simulink model "Quadcopter"  (R2018a)
settings: Solver=VariableStepAuto  StartTime=0.0  StopTime=30  RelTol=1e-3
undefined symbols (not defined in the file): sigbuilder_block
libraries: simulink x5
settings Model: Creator=Admin  LastModifiedBy=Admin

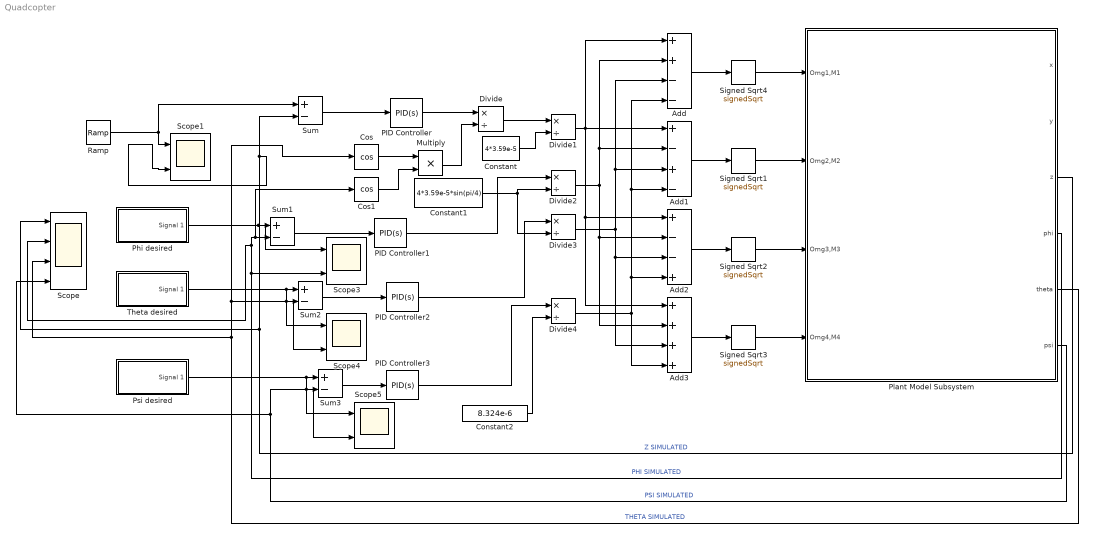
== system Quadcopter ==
  Add : Sum  Inputs=++--
  Add1 : Sum  Inputs=+-+-
  Add2 : Sum  Inputs=+--+
  Add3 : Sum  Inputs=++++
  Constant : Constant  Value=4*3.59e-5
  Constant1 : Constant  Value=4*3.59e-5*sin(pi/4)
  Constant2 : Constant  Value=8.324e-6
  Cos : Trigonometry  Operator=cos
  Cos1 : Trigonometry  Operator=cos
  Divide{,1..4} (5 alike) : Product  Inputs=*/
  Multiply : Product
  PID Controller : simulink/Continuous/PID Controller  Controller=PID  TimeDomain=Continuous-time  SampleTime=-1  IntegratorMethod=Forward Euler  FilterMethod=Forward Euler  Form=Parallel  UseFilter=on  ControllerParametersSource=internal  P=5.605  I=1.3  D=1.3  N=100  InitialConditionSource=internal  InitialConditionForIntegrator=0  InitialConditionForFilter=0  ExternalReset=none  LimitOutput=off  UpperSaturationLimit=inf  LowerSaturationLimit=-inf  LinearizeAsGain=on  AntiWindupMode=none  Kb=1  TrackingMode=off  Kt=1  PParamMin=[]  PParamMax=[]  IParamMin=[]  IParamMax=[]  DParamMin=[]  DParamMax=[]  NParamMin=[]  NParamMax=[]  KbParamMin=[]  KbParamMax=[]  KtParamMin=[]  KtParamMax=[]  POutMin=[]  POutMax=[]  IOutMin=[]  IOutMax=[]  DOutMin=[]  DOutMax=[]  NOutMin=[]  NOutMax=[]  KbOutMin=[]  KbOutMax=[]  KtOutMin=[]  KtOutMax=[]  IntegratorOutMin=[]  IntegratorOutMax=[]  FilterOutMin=[]  FilterOutMax=[]  SumOutMin=[]  SumOutMax=[]  SumI1OutMin=[]  SumI1OutMax=[]  SumI2OutMin=[]  SumI2OutMax=[]  SumI3OutMin=[]  SumI3OutMax=[]  SumDOutMin=[]  SumDOutMax=[]  SaturationOutMin=[]  SaturationOutMax=[]  IntegratorContinuousStateAttributes=''  IntegratorStateMustResolveToSignalObject=off  IntegratorRTWStateStorageClass=Auto  FilterContinuousStateAttributes=''  FilterStateMustResolveToSignalObject=off  FilterRTWStateStorageClass=Auto  DifferentiatorICPrevScaledInput=0  DifferentiatorOutMin=[]  DifferentiatorOutMax=[]  FilterDiffOutCoefMin=[]  FilterDiffOutCoefMax=[]  SumDenOutMin=[]  SumDenOutMax=[]  SumNumOutMin=[]  SumNumOutMax=[]  ReciprocalOutMin=[]  ReciprocalOutMax=[]  DivideOutMin=[]  DivideOutMax=[]  TunerSelectOption=Transfer Function Based (PID Tuner App)
  PID Controller1 : simulink/Continuous/PID Controller  Controller=PID  TimeDomain=Continuous-time  SampleTime=-1  IntegratorMethod=Forward Euler  FilterMethod=Forward Euler  Form=Parallel  UseFilter=on  ControllerParametersSource=internal  P=0.006  I=0.0001  D=0.2  N=100  InitialConditionSource=internal  InitialConditionForIntegrator=0  InitialConditionForFilter=0  ExternalReset=none  LimitOutput=off  UpperSaturationLimit=inf  LowerSaturationLimit=-inf  LinearizeAsGain=on  AntiWindupMode=none  Kb=1  TrackingMode=off  Kt=1  PParamMin=[]  PParamMax=[]  IParamMin=[]  IParamMax=[]  DParamMin=[]  DParamMax=[]  NParamMin=[]  NParamMax=[]  KbParamMin=[]  KbParamMax=[]  KtParamMin=[]  KtParamMax=[]  POutMin=[]  POutMax=[]  IOutMin=[]  IOutMax=[]  DOutMin=[]  DOutMax=[]  NOutMin=[]  NOutMax=[]  KbOutMin=[]  KbOutMax=[]  KtOutMin=[]  KtOutMax=[]  IntegratorOutMin=[]  IntegratorOutMax=[]  FilterOutMin=[]  FilterOutMax=[]  SumOutMin=[]  SumOutMax=[]  SumI1OutMin=[]  SumI1OutMax=[]  SumI2OutMin=[]  SumI2OutMax=[]  SumI3OutMin=[]  SumI3OutMax=[]  SumDOutMin=[]  SumDOutMax=[]  SaturationOutMin=[]  SaturationOutMax=[]  IntegratorContinuousStateAttributes=''  IntegratorStateMustResolveToSignalObject=off  IntegratorRTWStateStorageClass=Auto  FilterContinuousStateAttributes=''  FilterStateMustResolveToSignalObject=off  FilterRTWStateStorageClass=Auto  DifferentiatorICPrevScaledInput=0  DifferentiatorOutMin=[]  DifferentiatorOutMax=[]  FilterDiffOutCoefMin=[]  FilterDiffOutCoefMax=[]  SumDenOutMin=[]  SumDenOutMax=[]  SumNumOutMin=[]  SumNumOutMax=[]  ReciprocalOutMin=[]  ReciprocalOutMax=[]  DivideOutMin=[]  DivideOutMax=[]  TunerSelectOption=Transfer Function Based (PID Tuner App)
  PID Controller2 : simulink/Continuous/PID Controller  Controller=PID  TimeDomain=Continuous-time  SampleTime=-1  IntegratorMethod=Forward Euler  FilterMethod=Forward Euler  Form=Parallel  UseFilter=on  ControllerParametersSource=internal  P=0.006  I=0.0001  D=0.2  N=100  InitialConditionSource=internal  InitialConditionForIntegrator=0  InitialConditionForFilter=0  ExternalReset=none  LimitOutput=off  UpperSaturationLimit=inf  LowerSaturationLimit=-inf  LinearizeAsGain=on  AntiWindupMode=none  Kb=1  TrackingMode=off  Kt=1  PParamMin=[]  PParamMax=[]  IParamMin=[]  IParamMax=[]  DParamMin=[]  DParamMax=[]  NParamMin=[]  NParamMax=[]  KbParamMin=[]  KbParamMax=[]  KtParamMin=[]  KtParamMax=[]  POutMin=[]  POutMax=[]  IOutMin=[]  IOutMax=[]  DOutMin=[]  DOutMax=[]  NOutMin=[]  NOutMax=[]  KbOutMin=[]  KbOutMax=[]  KtOutMin=[]  KtOutMax=[]  IntegratorOutMin=[]  IntegratorOutMax=[]  FilterOutMin=[]  FilterOutMax=[]  SumOutMin=[]  SumOutMax=[]  SumI1OutMin=[]  SumI1OutMax=[]  SumI2OutMin=[]  SumI2OutMax=[]  SumI3OutMin=[]  SumI3OutMax=[]  SumDOutMin=[]  SumDOutMax=[]  SaturationOutMin=[]  SaturationOutMax=[]  IntegratorContinuousStateAttributes=''  IntegratorStateMustResolveToSignalObject=off  IntegratorRTWStateStorageClass=Auto  FilterContinuousStateAttributes=''  FilterStateMustResolveToSignalObject=off  FilterRTWStateStorageClass=Auto  DifferentiatorICPrevScaledInput=0  DifferentiatorOutMin=[]  DifferentiatorOutMax=[]  FilterDiffOutCoefMin=[]  FilterDiffOutCoefMax=[]  SumDenOutMin=[]  SumDenOutMax=[]  SumNumOutMin=[]  SumNumOutMax=[]  ReciprocalOutMin=[]  ReciprocalOutMax=[]  DivideOutMin=[]  DivideOutMax=[]  TunerSelectOption=Transfer Function Based (PID Tuner App)
  PID Controller3 : simulink/Continuous/PID Controller  Controller=PID  TimeDomain=Continuous-time  SampleTime=-1  IntegratorMethod=Forward Euler  FilterMethod=Forward Euler  Form=Parallel  UseFilter=on  ControllerParametersSource=internal  P=0.09  I=0.005  D=0.07  N=100  InitialConditionSource=internal  InitialConditionForIntegrator=0  InitialConditionForFilter=0  ExternalReset=none  LimitOutput=off  UpperSaturationLimit=inf  LowerSaturationLimit=-inf  LinearizeAsGain=on  AntiWindupMode=none  Kb=1  TrackingMode=off  Kt=1  PParamMin=[]  PParamMax=[]  IParamMin=[]  IParamMax=[]  DParamMin=[]  DParamMax=[]  NParamMin=[]  NParamMax=[]  KbParamMin=[]  KbParamMax=[]  KtParamMin=[]  KtParamMax=[]  POutMin=[]  POutMax=[]  IOutMin=[]  IOutMax=[]  DOutMin=[]  DOutMax=[]  NOutMin=[]  NOutMax=[]  KbOutMin=[]  KbOutMax=[]  KtOutMin=[]  KtOutMax=[]  IntegratorOutMin=[]  IntegratorOutMax=[]  FilterOutMin=[]  FilterOutMax=[]  SumOutMin=[]  SumOutMax=[]  SumI1OutMin=[]  SumI1OutMax=[]  SumI2OutMin=[]  SumI2OutMax=[]  SumI3OutMin=[]  SumI3OutMax=[]  SumDOutMin=[]  SumDOutMax=[]  SaturationOutMin=[]  SaturationOutMax=[]  IntegratorContinuousStateAttributes=''  IntegratorStateMustResolveToSignalObject=off  IntegratorRTWStateStorageClass=Auto  FilterContinuousStateAttributes=''  FilterStateMustResolveToSignalObject=off  FilterRTWStateStorageClass=Auto  DifferentiatorICPrevScaledInput=0  DifferentiatorOutMin=[]  DifferentiatorOutMax=[]  FilterDiffOutCoefMin=[]  FilterDiffOutCoefMax=[]  SumDenOutMin=[]  SumDenOutMax=[]  SumNumOutMin=[]  SumNumOutMax=[]  ReciprocalOutMin=[]  ReciprocalOutMax=[]  DivideOutMin=[]  DivideOutMax=[]  TunerSelectOption=Transfer Function Based (PID Tuner App)
  Phi desired : Subsystem  Tag=STV Subsys  LoadFcn=sigbuilder_block('load');  StartFcn=sigbuilder_block('start');  StopFcn=sigbuilder_block('stop');  ClipboardFcn=sigbuilder_block('clipboard');  mask(Sigbuilder block){tuvar=[0:10]}
      mask help: Simulink:masks:SigbuilderBlock_MD
      mask init:
      | if ~strcmp(get_param(bdroot(gcbh),'SimulationStatus'),'stopped') tuvar = sigbuilder_block('maskInit'); end
      settings: CopyFcn=sigbuilder_block('copy');  DeleteFcn=sigbuilder_block('delete');  ModelCloseFcn=sigbuilder_block('modelClose');  PreSaveFcn=sigbuilder_block('preSave');  PauseFcn=sigbuilder_block('pause');  ContinueFcn=sigbuilder_block('continue');  NameChangeFcn=sigbuilder_block('namechange');  OpenFcn=sigbuilder_block('open',[426.6 123.6 550.8 400.2 ]);  CloseFcn=sigbuilder_block('close');
      mask Display: plot(0, 0, 100, 100,[2, 2, 32, 32, 2], [68, 8, 8, 68, 68],[32, 2], [38, 38], [32, 19, 2],[53, 60, 44], [32, 17, 17, 2],[16, 16, 31, 31]);txt = getActiveGroup(gcbh);text(2, 100, txt,'verticalAlignment', 'top');
  Plant Model Subsystem : Subsystem
  Psi desired : Subsystem  Tag=STV Subsys  LoadFcn=sigbuilder_block('load');  StartFcn=sigbuilder_block('start');  StopFcn=sigbuilder_block('stop');  ClipboardFcn=sigbuilder_block('clipboard');  mask(Sigbuilder block){tuvar=[0:10]}
      mask help: Simulink:masks:SigbuilderBlock_MD
      mask init:
      | if ~strcmp(get_param(bdroot(gcbh),'SimulationStatus'),'stopped') tuvar = sigbuilder_block('maskInit'); end
      settings: CopyFcn=sigbuilder_block('copy');  DeleteFcn=sigbuilder_block('delete');  ModelCloseFcn=sigbuilder_block('modelClose');  PreSaveFcn=sigbuilder_block('preSave');  PauseFcn=sigbuilder_block('pause');  ContinueFcn=sigbuilder_block('continue');  NameChangeFcn=sigbuilder_block('namechange');  OpenFcn=sigbuilder_block('open',[426.6 123.6 550.8 400.2 ]);  CloseFcn=sigbuilder_block('close');
      mask Display: plot(0, 0, 100, 100,[2, 2, 32, 32, 2], [68, 8, 8, 68, 68],[32, 2], [38, 38], [32, 19, 2],[53, 60, 44], [32, 17, 17, 2],[16, 16, 31, 31]);txt = getActiveGroup(gcbh);text(2, 100, txt,'verticalAlignment', 'top');
  Ramp : simulink/Sources/Ramp  slope=1.5  start=0  InitialOutput=0
  Scope : Scope  NumInputPorts=4
  Scope{1,3..5} (4 alike) : Scope  NumInputPorts=2
  Signed Sqrt{1..4} (4 alike) : Sqrt  Operator=signedSqrt  SaturateOnIntegerOverflow=on
  Sum{,1..3} (4 alike) : Sum  Inputs=+-
  Theta desired : Subsystem  Tag=STV Subsys  LoadFcn=sigbuilder_block('load');  StartFcn=sigbuilder_block('start');  StopFcn=sigbuilder_block('stop');  ClipboardFcn=sigbuilder_block('clipboard');  mask(Sigbuilder block){tuvar=[0:10]}
      mask help: Simulink:masks:SigbuilderBlock_MD
      mask init:
      | if ~strcmp(get_param(bdroot(gcbh),'SimulationStatus'),'stopped') tuvar = sigbuilder_block('maskInit'); end
      settings: CopyFcn=sigbuilder_block('copy');  DeleteFcn=sigbuilder_block('delete');  ModelCloseFcn=sigbuilder_block('modelClose');  PreSaveFcn=sigbuilder_block('preSave');  PauseFcn=sigbuilder_block('pause');  ContinueFcn=sigbuilder_block('continue');  NameChangeFcn=sigbuilder_block('namechange');  OpenFcn=sigbuilder_block('open',[426.6 123.6 550.8 400.2 ]);  CloseFcn=sigbuilder_block('close');
      mask Display: plot(0, 0, 100, 100,[2, 2, 32, 32, 2], [68, 8, 8, 68, 68],[32, 2], [38, 38], [32, 19, 2],[53, 60, 44], [32, 17, 17, 2],[16, 16, 31, 31]);txt = getActiveGroup(gcbh);text(2, 100, txt,'verticalAlignment', 'top');
  wires:
  Sum/1 -> PID Controller/1
  PID Controller/1 -> Divide/1
  Multiply/1 -> Divide/2
  Cos/1 -> Multiply/1
  Cos1/1 -> Multiply/2
  Sum1/1 -> PID Controller1/1
  Sum2/1 -> PID Controller2/1
  Sum3/1 -> PID Controller3/1
  Psi desired/1(Signal 1) -> Scope5/1, Sum3/1
  Theta desired/1(Signal 1) -> Scope4/1, Sum2/1
  Phi desired/1(Signal 1) -> Scope3/1, Sum1/1
  Plant Model Subsystem/3(z) -> Scope1/2, Sum/2, Scope/1  "Z SIMULATED"
  Plant Model Subsystem/4(phi) -> Scope3/2, Scope/2, Sum1/2, Cos1/1  "PHI SIMULATED"
  Plant Model Subsystem/5(theta) -> Cos/1, Scope4/2, Sum2/2, Scope/3  "THETA SIMULATED"
  Plant Model Subsystem/6(psi) -> Scope5/2, Sum3/2, Scope/4  "PSI SIMULATED"
  Divide/1 -> Divide1/1
  PID Controller1/1 -> Divide2/1
  PID Controller2/1 -> Divide3/1
  PID Controller3/1 -> Divide4/1
  Constant2/1 -> Divide4/2
  Divide1/1 -> Add3/1, Add2/1, Add1/1, Add/1
  Divide2/1 -> Add3/2, Add2/2, Add1/2, Add/2
  Divide3/1 -> Add3/3, Add2/3, Add/3, Add1/3
  Divide4/1 -> Add3/4, Add1/4, Add/4, Add2/4
  Add1/1 -> Signed Sqrt1/1
  Add2/1 -> Signed Sqrt2/1
  Add3/1 -> Signed Sqrt3/1
  Add/1 -> Signed Sqrt4/1
  Constant/1 -> Divide1/2
  Signed Sqrt4/1 -> Plant Model Subsystem/1(Omg1,M1)
  Signed Sqrt1/1 -> Plant Model Subsystem/2(Omg2,M2)
  Signed Sqrt2/1 -> Plant Model Subsystem/3(Omg3,M3)
  Signed Sqrt3/1 -> Plant Model Subsystem/4(Omg4,M4)
  Constant1/1 -> Divide2/2, Divide3/2
  Ramp/1 -> Sum/1, Scope1/1

== system Quadcopter/Phi desired ==
  Demux : Demux  Tag=STV Demux  Outputs=1
  FromWs : FromWorkspace  Tag=STV FromWs  VariableName=tuvar  SampleTime=0
      SigBuilderData=|
      | common.afterFinalStr = 'Extrapolate'
      | common.sampleTime = 0
      | dataSet.timeRange = [0 10]
      | dataSet.name = 'Group 1'
      | sbobj.Groups.Name = 'Group 1'
      | sbobj.Groups.Signals.Name = 'Signal 1'
      | sbobj.Groups.Signals.XData = [0 4 4 7 7 10]
      | sbobj.Groups.Signals.YData = [0 0 0.198 0.198 0.001 0]
  Signal 1 : Outport  Tag=STV Outport
  wires:
  Demux/1 -> Signal 1/1
  FromWs/1 -> Demux/1

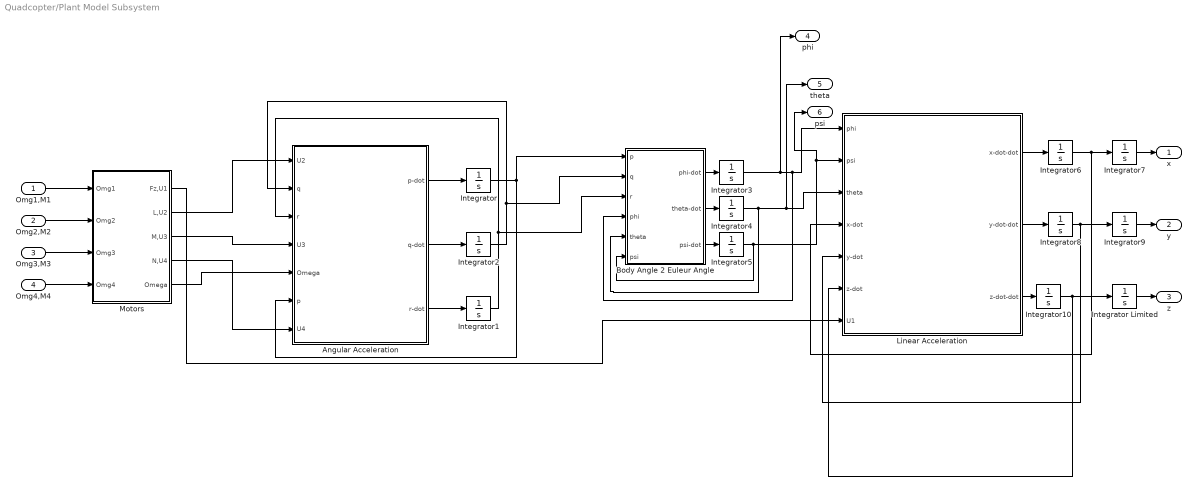
== system Quadcopter/Plant Model Subsystem ==
  Omg1,M1 : Inport
  Omg2,M2 : Inport  Port=2
  Omg3,M3 : Inport  Port=3
  Omg4,M4 : Inport  Port=4
  Angular Acceleration : Subsystem  mask{Jr=0, Ixx=0.00963, Iyy=0.00963, Izz=0.019}
  Body Angle 2 Euleur Angle : Subsystem
  Integrator{,1..2,6..10} (8 alike) : Integrator
  Integrator Limited : Integrator  LimitOutput=on  UpperSaturationLimit=1000  LowerSaturationLimit=0
  Integrator3 : Integrator  WrapState=on
  Integrator4 : Integrator  WrapState=on
  Integrator5 : Integrator  WrapState=on
  Linear Acceleration : Subsystem  mask{Kd=0.1, g=9.81, m=0.9928}
      mask prompts: g "Gia toc trong truong g(m/s2)"; m "Khoi luong m (kg)"
  Motors : Subsystem  mask{b=3.59e-5, d=2.0810e-6}
  x : Outport
  y : Outport  Port=2
  z : Outport  Port=3
  phi : Outport  Port=4
  theta : Outport  Port=5
  psi : Outport  Port=6
  wires:
  Omg4,M4/1 -> Motors/4(Omg4)
  Omg3,M3/1 -> Motors/3(Omg3)
  Omg2,M2/1 -> Motors/2(Omg2)
  Omg1,M1/1 -> Motors/1(Omg1)
  Motors/2(L,U2) -> Angular Acceleration/1(U2)
  Motors/3(M,U3) -> Angular Acceleration/4(U3)
  Motors/4(N,U4) -> Angular Acceleration/7(U4)
  Motors/5(Omega) -> Angular Acceleration/5(Omega)
  Angular Acceleration/1(p-dot) -> Integrator/1
  Angular Acceleration/2(q-dot) -> Integrator2/1
  Angular Acceleration/3(r-dot) -> Integrator1/1
  Integrator/1 -> Body Angle 2 Euleur Angle/1(p), Angular Acceleration/6(p)
  Integrator2/1 -> Body Angle 2 Euleur Angle/2(q), Angular Acceleration/2(q)
  Integrator3/1 -> phi/1, Body Angle 2 Euleur Angle/4(phi), Linear Acceleration/1(phi)
  Integrator4/1 -> Body Angle 2 Euleur Angle/5(theta), theta/1, Linear Acceleration/3(theta)
  Integrator1/1 -> Body Angle 2 Euleur Angle/3(r), Angular Acceleration/3(r)
  Integrator5/1 -> Body Angle 2 Euleur Angle/6(psi), psi/1, Linear Acceleration/2(psi)
  Integrator6/1 -> Linear Acceleration/4(x-dot), Integrator7/1
  Integrator7/1 -> x/1
  Integrator8/1 -> Linear Acceleration/5(y-dot), Integrator9/1
  Integrator9/1 -> y/1
  Integrator10/1 -> Integrator Limited/1, Linear Acceleration/6(z-dot)
  Integrator Limited/1 -> z/1
  Linear Acceleration/3(z-dot-dot) -> Integrator10/1
  Linear Acceleration/2(y-dot-dot) -> Integrator8/1
  Linear Acceleration/1(x-dot-dot) -> Integrator6/1
  Motors/1(Fz,U1) -> Linear Acceleration/7(U1)
  Body Angle 2 Euleur Angle/1(phi-dot) -> Integrator3/1
  Body Angle 2 Euleur Angle/2(theta-dot) -> Integrator4/1
  Body Angle 2 Euleur Angle/3(psi-dot) -> Integrator5/1

== system Quadcopter/Psi desired ==
  Demux : Demux  Tag=STV Demux  Outputs=1
  FromWs : FromWorkspace  Tag=STV FromWs  VariableName=tuvar  SampleTime=0
      SigBuilderData=|
      | common.afterFinalStr = 'Extrapolate'
      | common.sampleTime = 0
      | dataSet.timeRange = [0 10]
      | dataSet.name = 'Group 1'
      | sbobj.Groups.Name = 'Group 1'
      | sbobj.Groups.Signals.Name = 'Signal 1'
      | sbobj.Groups.Signals.XData = [0 6.26 6.26 9.64 9.64 10]
      | sbobj.Groups.Signals.YData = [0 0 0.336 0.336 0 0]
  Signal 1 : Outport  Tag=STV Outport
  wires:
  Demux/1 -> Signal 1/1
  FromWs/1 -> Demux/1

== system Quadcopter/Theta desired ==
  Demux : Demux  Tag=STV Demux  Outputs=1
  FromWs : FromWorkspace  Tag=STV FromWs  VariableName=tuvar  SampleTime=0
      SigBuilderData=|
      | common.afterFinalStr = 'Extrapolate'
      | common.sampleTime = 0
      | dataSet.timeRange = [0 10]
      | dataSet.name = 'Group 1'
      | sbobj.Groups.Name = 'Group 1'
      | sbobj.Groups.Signals.Name = 'Signal 1'
      | sbobj.Groups.Signals.XData = [0 6.98 6.98 9 9 10]
      | sbobj.Groups.Signals.YData = [0 0 0.384 0.384 0 0]
  Signal 1 : Outport  Tag=STV Outport
  wires:
  Demux/1 -> Signal 1/1
  FromWs/1 -> Demux/1

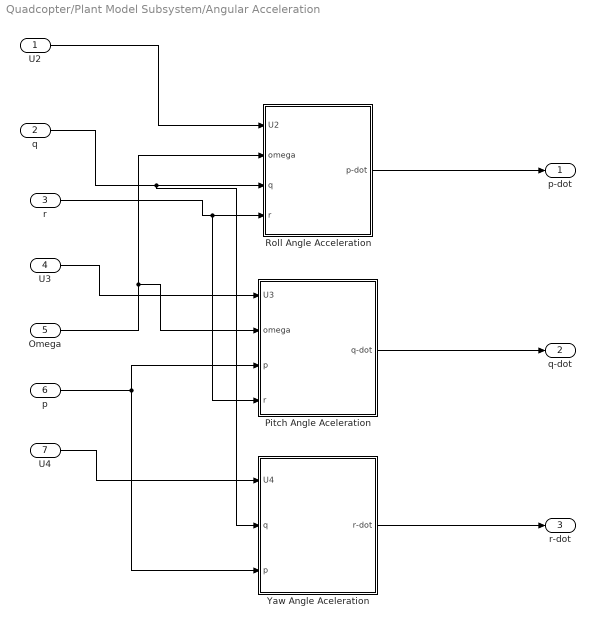
== system Quadcopter/Plant Model Subsystem/Angular Acceleration ==
  U2 : Inport
  q : Inport  Port=2
  r : Inport  Port=3
  U3 : Inport  Port=4
  Omega : Inport  Port=5
  p : Inport  Port=6
  U4 : Inport  Port=7
  Pitch Angle Aceleration : Subsystem
  Roll Angle Acceleration : Subsystem
  Yaw Angle Aceleration : Subsystem
  p-dot : Outport
  q-dot : Outport  Port=2
  r-dot : Outport  Port=3
  wires:
  Roll Angle Acceleration/1(p-dot) -> p-dot/1
  Pitch Angle Aceleration/1(q-dot) -> q-dot/1
  Yaw Angle Aceleration/1(r-dot) -> r-dot/1
  U2/1 -> Roll Angle Acceleration/1(U2)
  Omega/1 -> Pitch Angle Aceleration/2(omega), Roll Angle Acceleration/2(omega)
  U3/1 -> Pitch Angle Aceleration/1(U3)
  r/1 -> Pitch Angle Aceleration/4(r), Roll Angle Acceleration/4(r)
  p/1 -> Yaw Angle Aceleration/3(p), Pitch Angle Aceleration/3(p)
  U4/1 -> Yaw Angle Aceleration/1(U4)
  q/1 -> Yaw Angle Aceleration/2(q), Roll Angle Acceleration/3(q)

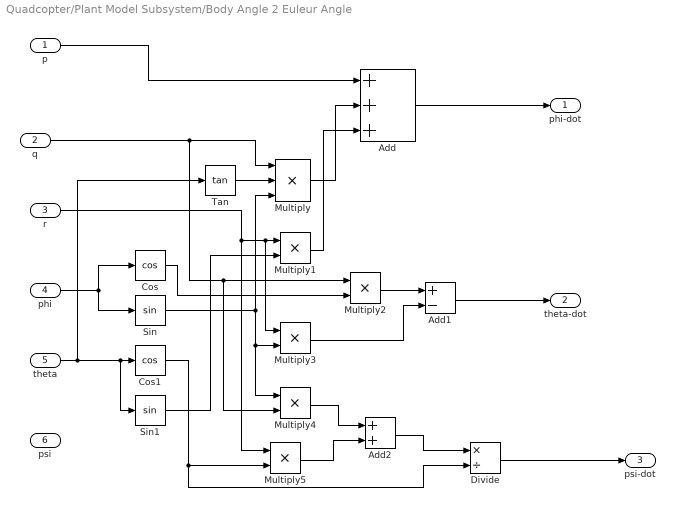
== system Quadcopter/Plant Model Subsystem/Body Angle 2 Euleur Angle ==
  p : Inport
  q : Inport  Port=2
  r : Inport  Port=3
  phi : Inport  Port=4
  theta : Inport  Port=5
  psi : Inport  Port=6
  Add : Sum  Inputs=+++
  Add1 : Sum  Inputs=+-
  Add2 : Sum
  Cos : Trigonometry  Operator=cos
  Cos1 : Trigonometry  Operator=cos
  Divide : Product  Inputs=*/
  Multiply : Product  Inputs=3
  Multiply{1..5} (5 alike) : Product
  Sin : Trigonometry
  Sin1 : Trigonometry
  Tan : Trigonometry  Operator=tan
  phi-dot : Outport
  theta-dot : Outport  Port=2
  psi-dot : Outport  Port=3
  wires:
  phi/1 -> Sin/1, Cos/1
  p/1 -> Add/1
  Tan/1 -> Multiply/2
  Sin/1 -> Multiply3/2, Multiply4/1, Multiply/3
  theta/1 -> Tan/1, Sin1/1, Cos1/1
  q/1 -> Multiply/1, Multiply4/2, Multiply2/1
  Multiply/1 -> Add/2
  r/1 -> Multiply5/1, Multiply3/1, Multiply1/1
  Sin1/1 -> Multiply1/2
  Multiply1/1 -> Add/3
  Add/1 -> phi-dot/1
  Cos/1 -> Multiply2/2
  Multiply2/1 -> Add1/1
  Multiply3/1 -> Add1/2
  Add1/1 -> theta-dot/1
  Cos1/1 -> Divide/2, Multiply5/2
  Multiply5/1 -> Add2/2
  Multiply4/1 -> Add2/1
  Add2/1 -> Divide/1
  Divide/1 -> psi-dot/1

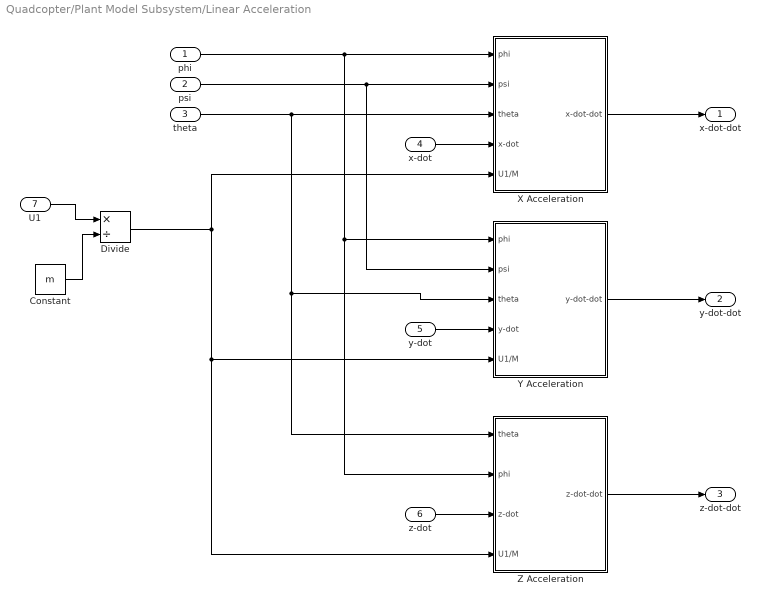
== system Quadcopter/Plant Model Subsystem/Linear Acceleration ==
  phi : Inport
  psi : Inport  Port=2
  theta : Inport  Port=3
  x-dot : Inport  Port=4
  y-dot : Inport  Port=5
  z-dot : Inport  Port=6
  U1 : Inport  Port=7
  Constant : Constant  Value=m
  Divide : Product  Inputs=*/
  X Acceleration : Subsystem
  Y Acceleration : Subsystem
  Z Acceleration : Subsystem
  x-dot-dot : Outport
  y-dot-dot : Outport  Port=2
  z-dot-dot : Outport  Port=3
  wires:
  phi/1 -> Z Acceleration/2(phi), Y Acceleration/1(phi), X Acceleration/1(phi)
  psi/1 -> Y Acceleration/2(psi), X Acceleration/2(psi)
  theta/1 -> Y Acceleration/3(theta), Z Acceleration/1(theta), X Acceleration/3(theta)
  x-dot/1 -> X Acceleration/4(x-dot)
  y-dot/1 -> Y Acceleration/4(y-dot)
  z-dot/1 -> Z Acceleration/3(z-dot)
  U1/1 -> Divide/1
  Constant/1 -> Divide/2
  Divide/1 -> Z Acceleration/4(U1/M), Y Acceleration/5(U1/M), X Acceleration/5(U1/M)
  X Acceleration/1(x-dot-dot) -> x-dot-dot/1
  Y Acceleration/1(y-dot-dot) -> y-dot-dot/1
  Z Acceleration/1(z-dot-dot) -> z-dot-dot/1

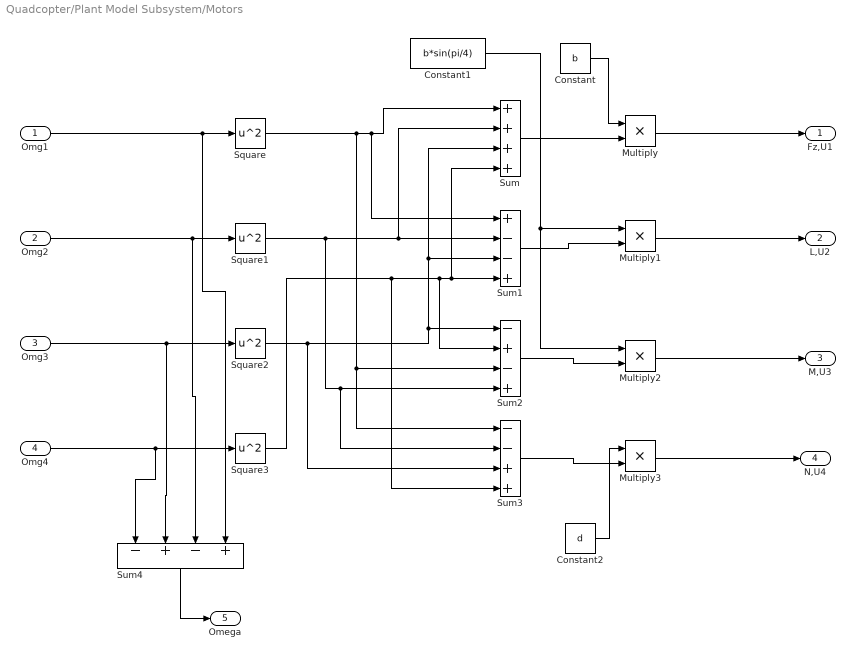
== system Quadcopter/Plant Model Subsystem/Motors ==
  Omg1 : Inport
  Omg2 : Inport  Port=2
  Omg3 : Inport  Port=3
  Omg4 : Inport  Port=4
  Constant : Constant  Value=b
  Constant1 : Constant  Value=b*sin(pi/4)
  Constant2 : Constant  Value=d
  Multiply{,1..3} (4 alike) : Product
  Square{,1..3} (4 alike) : Math  Operator=square  SaturateOnIntegerOverflow=on
  Sum : Sum  Inputs=++++
  Sum1 : Sum  Inputs=+--+
  Sum2 : Sum  Inputs=-+-+
  Sum3 : Sum  Inputs=--++
  Sum4 : Sum  Inputs=-+-+
  Fz,U1 : Outport
  L,U2 : Outport  Port=2
  M,U3 : Outport  Port=3
  N,U4 : Outport  Port=4
  Omega : Outport  Port=5
  wires:
  Square/1 -> Sum3/1, Sum2/3, Sum1/1, Sum/1
  Square1/1 -> Sum3/2, Sum2/4, Sum/2, Sum1/2
  Square2/1 -> Sum3/3, Sum2/1, Sum/3, Sum1/3
  Square3/1 -> Sum3/4, Sum2/2, Sum/4, Sum1/4
  Sum/1 -> Multiply/2
  Sum1/1 -> Multiply1/2
  Sum2/1 -> Multiply2/2
  Sum3/1 -> Multiply3/2
  Constant/1 -> Multiply/1
  Constant1/1 -> Multiply2/1, Multiply1/1
  Constant2/1 -> Multiply3/1
  Multiply/1 -> Fz,U1/1
  Multiply1/1 -> L,U2/1
  Multiply2/1 -> M,U3/1
  Multiply3/1 -> N,U4/1
  Omg1/1 -> Sum4/4, Square/1
  Omg2/1 -> Sum4/3, Square1/1
  Omg3/1 -> Sum4/2, Square2/1
  Omg4/1 -> Sum4/1, Square3/1
  Sum4/1 -> Omega/1

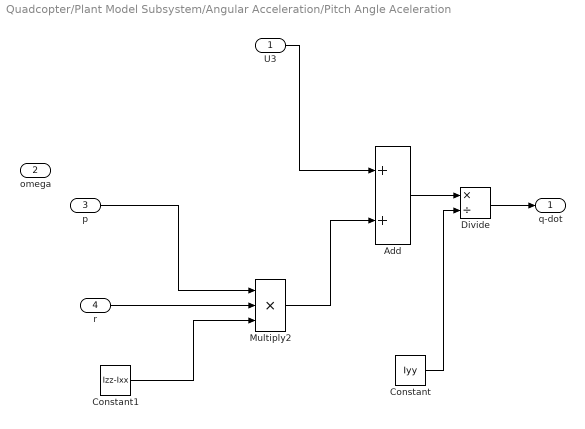
== system Quadcopter/Plant Model Subsystem/Angular Acceleration/Pitch Angle Aceleration ==
  U3 : Inport
  omega : Inport  Port=2
  p : Inport  Port=3
  r : Inport  Port=4
  Add : Sum
  Constant : Constant  Value=Iyy
  Constant1 : Constant  Value=Izz-Ixx
  Divide : Product  Inputs=*/
  Multiply2 : Product  Inputs=3
  q-dot : Outport
  wires:
  U3/1 -> Add/1
  Divide/1 -> q-dot/1
  r/1 -> Multiply2/2
  Constant1/1 -> Multiply2/3
  p/1 -> Multiply2/1
  Multiply2/1 -> Add/2
  Add/1 -> Divide/1
  Constant/1 -> Divide/2

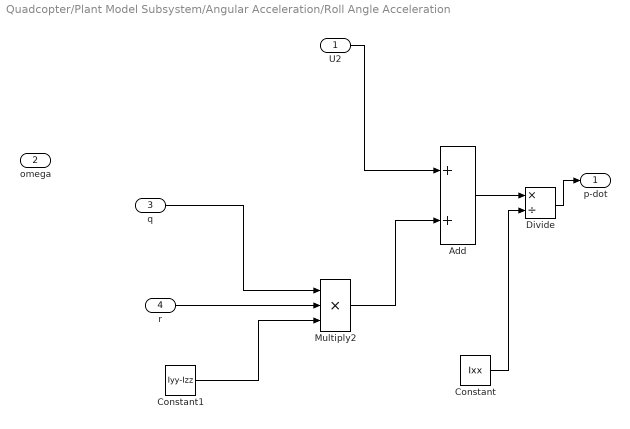
== system Quadcopter/Plant Model Subsystem/Angular Acceleration/Roll Angle Acceleration ==
  U2 : Inport
  omega : Inport  Port=2
  q : Inport  Port=3
  r : Inport  Port=4
  Add : Sum
  Constant : Constant  Value=Ixx
  Constant1 : Constant  Value=Iyy-Izz
  Divide : Product  Inputs=*/
  Multiply2 : Product  Inputs=3
  p-dot : Outport
  wires:
  U2/1 -> Add/1
  Divide/1 -> p-dot/1
  r/1 -> Multiply2/2
  Constant1/1 -> Multiply2/3
  q/1 -> Multiply2/1
  Multiply2/1 -> Add/2
  Add/1 -> Divide/1
  Constant/1 -> Divide/2

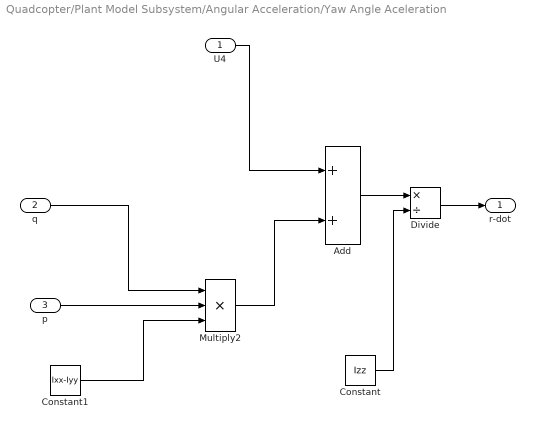
== system Quadcopter/Plant Model Subsystem/Angular Acceleration/Yaw Angle Aceleration ==
  U4 : Inport
  q : Inport  Port=2
  p : Inport  Port=3
  Add : Sum
  Constant : Constant  Value=Izz
  Constant1 : Constant  Value=Ixx-Iyy
  Divide : Product  Inputs=*/
  Multiply2 : Product  Inputs=3
  r-dot : Outport
  wires:
  U4/1 -> Add/1
  Divide/1 -> r-dot/1
  p/1 -> Multiply2/2
  Constant1/1 -> Multiply2/3
  q/1 -> Multiply2/1
  Multiply2/1 -> Add/2
  Add/1 -> Divide/1
  Constant/1 -> Divide/2

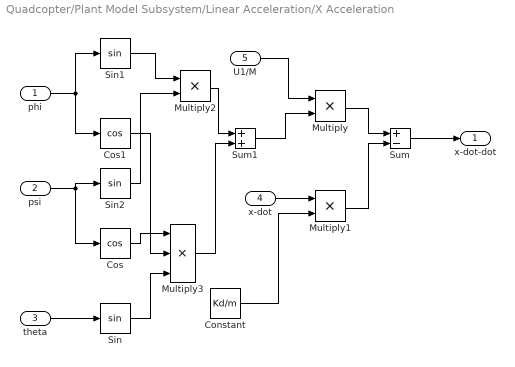
== system Quadcopter/Plant Model Subsystem/Linear Acceleration/X Acceleration ==
  phi : Inport
  psi : Inport  Port=2
  theta : Inport  Port=3
  x-dot : Inport  Port=4
  U1/M : Inport  Port=5
  Constant : Constant  Value=Kd/m
  Cos : Trigonometry  Operator=cos
  Cos1 : Trigonometry  Operator=cos
  Multiply : Product
  Multiply1 : Product
  Multiply2 : Product
  Multiply3 : Product  Inputs=3
  Sin : Trigonometry
  Sin1 : Trigonometry
  Sin2 : Trigonometry
  Sum : Sum  Inputs=+-
  Sum1 : Sum
  x-dot-dot : Outport
  wires:
  Sum/1 -> x-dot-dot/1
  x-dot/1 -> Multiply1/1
  Constant/1 -> Multiply1/2
  Multiply1/1 -> Sum/2
  Multiply/1 -> Sum/1
  theta/1 -> Sin/1
  phi/1 -> Cos1/1, Sin1/1
  psi/1 -> Cos/1, Sin2/1
  Sin/1 -> Multiply3/3
  Cos1/1 -> Multiply3/2
  Cos/1 -> Multiply3/1
  Sin2/1 -> Multiply2/2
  Sin1/1 -> Multiply2/1
  Multiply2/1 -> Sum1/1
  Multiply3/1 -> Sum1/2
  Sum1/1 -> Multiply/2
  U1/M/1 -> Multiply/1

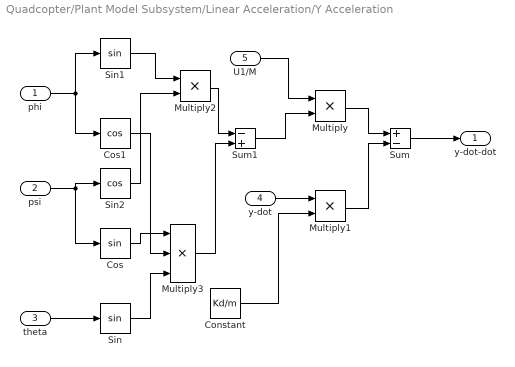
== system Quadcopter/Plant Model Subsystem/Linear Acceleration/Y Acceleration ==
  phi : Inport
  psi : Inport  Port=2
  theta : Inport  Port=3
  y-dot : Inport  Port=4
  U1/M : Inport  Port=5
  Constant : Constant  Value=Kd/m
  Cos : Trigonometry
  Cos1 : Trigonometry  Operator=cos
  Multiply : Product
  Multiply1 : Product
  Multiply2 : Product
  Multiply3 : Product  Inputs=3
  Sin : Trigonometry
  Sin1 : Trigonometry
  Sin2 : Trigonometry  Operator=cos
  Sum : Sum  Inputs=+-
  Sum1 : Sum  Inputs=-+
  y-dot-dot : Outport
  wires:
  Sum/1 -> y-dot-dot/1
  y-dot/1 -> Multiply1/1
  Constant/1 -> Multiply1/2
  Multiply1/1 -> Sum/2
  Multiply/1 -> Sum/1
  theta/1 -> Sin/1
  phi/1 -> Cos1/1, Sin1/1
  psi/1 -> Cos/1, Sin2/1
  Sin/1 -> Multiply3/3
  Cos1/1 -> Multiply3/2
  Cos/1 -> Multiply3/1
  Sin2/1 -> Multiply2/2
  Sin1/1 -> Multiply2/1
  Multiply2/1 -> Sum1/1
  Multiply3/1 -> Sum1/2
  Sum1/1 -> Multiply/2
  U1/M/1 -> Multiply/1

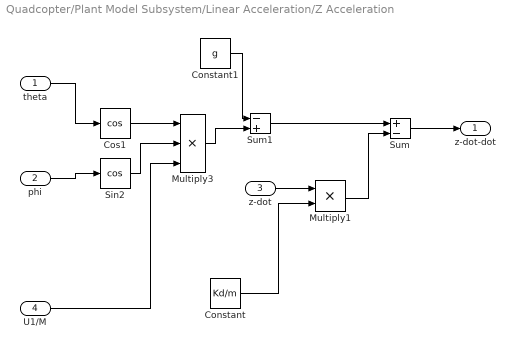
== system Quadcopter/Plant Model Subsystem/Linear Acceleration/Z Acceleration ==
  theta : Inport
  phi : Inport  Port=2
  z-dot : Inport  Port=3
  U1/M : Inport  Port=4
  Constant : Constant  Value=Kd/m
  Constant1 : Constant  Value=g
  Cos1 : Trigonometry  Operator=cos
  Multiply1 : Product
  Multiply3 : Product  Inputs=3
  Sin2 : Trigonometry  Operator=cos
  Sum : Sum  Inputs=+-
  Sum1 : Sum  Inputs=-+
  z-dot-dot : Outport
  wires:
  Sum/1 -> z-dot-dot/1
  z-dot/1 -> Multiply1/1
  Constant/1 -> Multiply1/2
  Multiply1/1 -> Sum/2
  Sum1/1 -> Sum/1
  theta/1 -> Cos1/1
  phi/1 -> Sin2/1
  U1/M/1 -> Multiply3/3
  Constant1/1 -> Sum1/1
  Multiply3/1 -> Sum1/2
  Cos1/1 -> Multiply3/1
  Sin2/1 -> Multiply3/2
